simulink model "ddc_bpm_476_066"  (Simulink 7.8)
settings: Solver=ode45  StartTime=0.0  StopTime=0.012  RelTol=1e-3
undefined symbols (not defined in the file): dt_sim, frev_476, Fs_adc, xlipgetpartsetting
libraries: xbsIndex_r4 x601, simulink x5
(part 1 of 6)
settings Model: Creator=lucas.russo  LastModifiedBy=lucas.russo
settings HardwareCC: ProdHWDeviceType=ASIC/FPGA->ASIC/FPGA  TargetIntDivRoundTo=Zero  TargetEndianess=LittleEndian  TargetHWDeviceType=MATLAB Host  ProdEqTarget=off

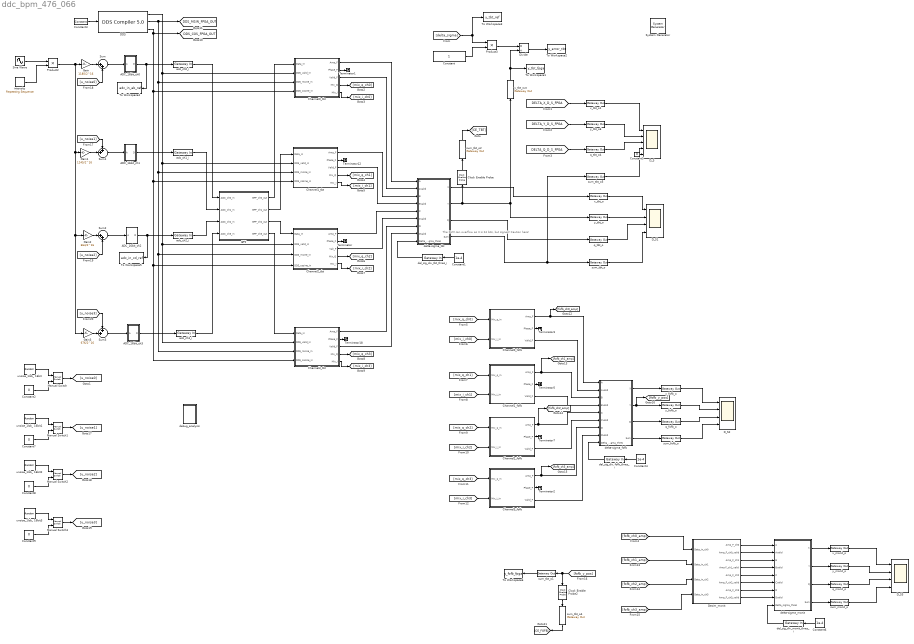
== system ddc_bpm_476_066 ==
  note: The SUM can overflow as it is 24 bits, but signed!
      | Caution here!
  " System Generator" : xbsIndex_r4/ System Generator  Tag=genX  xilinxfamily=virtex6  part=xc6vlx240t  speed=-1  package=ff1156  synthesis_tool=XST  clock_wrapper=Clock Enables  directory=./netlist_ddc_bpm_476_066  proj_type=Project Navigator  Synth_file=XST Defaults  Impl_file=ISE Defaults  testbench=off  simulink_period=dt_sim  sysclk_period=1/Fs_adc*1e9  dcm_input_clock_period=10  incr_netlist=off  trim_vbits=Everywhere in SubSystem  dbl_ovrd=According to Block Masks  core_generation=According to Block Masks  run_coregen=off  deprecated_control=off  eval_field=0  block_type=sysgen
  ADC_16bit_ch0 : Subsystem
  ADC_16bit_ch1 : Subsystem
  ADC_16bit_ch2 : Subsystem
  ADC_16bit_ch3 : Subsystem
  BPF : Subsystem
  Channel0_fofb : Subsystem
  Channel0_tbt : Subsystem
  Channel1_fofb : Subsystem
  Channel1_tbt : Subsystem
  Channel2_fofb : Subsystem
  Channel2_tbt : Subsystem
  Channel3_fofb : Subsystem
  Channel3_tbt : Subsystem
  Clock Enable Probe : xbsIndex_r4/Clock Enable Probe  inherit_constraints=on  block_type=ceprobe
      settings: infoedit="Clock enable extractor.  Produces a Boolean output that mirrors the hardware clock enable associated with the input sample rate.<br><br>Hardware notes: in hardware this block costs nothing."
  Clock Enable Probe2 : xbsIndex_r4/Clock Enable Probe  inherit_constraints=on  block_type=ceprobe
      settings: infoedit="Clock enable extractor.  Produces a Boolean output that mirrors the hardware clock enable associated with the input sample rate.<br><br>Hardware notes: in hardware this block costs nothing."
  Constant : Constant
  Constant1 : Constant  Value=1e-4  OutDataTypeStr=fixdt(1,26,22)
  Constant{2,7..9} (4 alike) : Constant  Value=0  SampleTime=0
  Constant3 : xbsIndex_r4/Constant  const=1  gui_display_data_type=Boolean  arith_type=Boolean  n_bits=24  bin_pt=22  preci_type=Single  exp_width=8  frac_width=24  explicit_period=on  period=dt_sim  equ=P=C  opselect=C  inp2=PCIN>>17  opr=+  inp1=P  carry=CIN  dbl_ovrd=off  block_type=constant
  Constant4 : Constant  Value=1e-4  OutDataTypeStr=fixdt(1,26,22)
  Constant5 : Constant  Value=0
  Constant6 : Constant  Value=1e-4  OutDataTypeStr=fixdt(1,26,22)
  DDS : xbsIndex_r4/DDS Compiler 5.0   partspresent=Phase_Generator_and_SIN_COS_LUT  dds_clock_rate=Fs_adc/1e6  channels=1  parameter_entry=Hardware_Parameters  spurious_free_dynamic_range=36  frequency_resolution=0.4  noise_shaping=Taylor_Series_Corrected  phase_width=30  output_width=24  output_selection=Sine_and_Cosine  negative_sine=on  negative_cosine=off  amplitude_mode=Unit_Circle  memory_type=Auto  optimization_goal=Auto  dsp48_use=Minimal  latency_configuration=Auto  latency=10  has_phase_out=off  has_aclken=off  has_aresetn=off  explicit_period=on  period=dt_sim  data_has_tlast=Not_Required  has_tready=on  s_phase_has_tuser=Not_Required  m_data_has_tuser=Not_Required  m_phase_has_tuser=Not_Required  s_phase_tuser_width=1  s_config_sync_mode=On_Vector  phase_increment=Fixed  output_frequency1=0  output_frequency2=0  output_frequency3=0  output_frequency4=0  output_frequency5=0  output_frequency6=0  output_frequency7=0  output_frequency8=0  output_frequency9=0  output_frequency10=0  output_frequency11=0  output_frequency12=0  output_frequency13=0  output_frequency14=0  output_frequency15=0  output_frequency16=0  pinc1=dds_freq_bin  pinc2='0'  pinc3='0'  pinc4='0'  pinc5='0'  pinc6='0'  pinc7='0'  pinc8='0'  pinc9='0'  pinc10='0'  pinc11='0'  pinc12='0'  pinc13='0'  pinc14='0'  pinc15='0'  pinc16='0'  phase_offset=Fixed  phase_offset_angles1=0  phase_offset_angles2=0  phase_offset_angles3=0  phase_offset_angles4=0  phase_offset_angles5=0  phase_offset_angles6=0  phase_offset_angles7=0  phase_offset_angles8=0  phase_offset_angles9=0  phase_offset_angles10=0  phase_offset_angles11=0  phase_offset_angles12=0  phase_offset_angles13=0  phase_offset_angles14=0  phase_offset_angles15=0  phase_offset_angles16=0  poff1='0'  poff2='0'  poff3='0'  poff4='0'  poff5='0'  poff6='0'  poff7='0'  poff8='0'  poff9='0'  poff10='0'  poff11='0'  poff12='0'  poff13='0'  poff14='0'  poff15='0'  poff16='0'  trim_axipin_name=on  por_mode=false  gui_behaviour=Sysgen  ip_name=DDS Compiler  ip_version=5.0  dsptool_ready=true  wrapper_available=true  port_translation_map={ 'aclken' => 'en', 'aresetn' => 'rst' }  ipcore_xco_need_fpga_part=true  ipcore_fpga_part=xlipgetpartsetting(gcb, {'virtex6', 'xc6vlx75t', '-3', 'ff784'})  ipcore_usecache=true  ipcore_useipmodelcache=true  ipcore_verbose=false  block_type=dds_compiler_v5_0
  D_S : Scope  NumInputPorts=5
      settings: TimeRange=0.0004  YMin=-1~0~10~0~0  YMax=1~0.00025~100~2.5~1  SaveName=ScopeData7  MaxDataPoints=1000000  SampleInput=on
  D_S1 : Scope  NumInputPorts=4
      settings: TimeRange=0.0003  YMin=-1~-1~-1~0.0190031  YMax=1~1~1~0.0210035  SaveName=ScopeData6  MaxDataPoints=1000000  SampleInput=on
  D_S2 : Scope  NumInputPorts=4
      settings: TimeRange=0.002999999999999999  YMin=-1~-1~-1~0.0190031  YMax=1~1~1~0.0210035  SaveName=ScopeData11  MaxDataPoints=1000000  SampleInput=on
  D_S3 : Scope  NumInputPorts=4
      settings: TimeRange=0.0003  YMin=-1~-1~-1~0.0190031  YMax=1~1~1~0.0210035  SaveName=ScopeData12  MaxDataPoints=1000000  SampleInput=on
  Decim_monit : Subsystem
  Divide : Product  Inputs=*/
  Gain : Gain  Gain=1185/2^16
  Gain1 : Gain  Gain=1245/2^16
  Gain2 : Gain  Gain=664/2^16
  Gain3 : Gain  Gain=676/2^16
  Manual Switch{,1..3} (4 alike) : simulink/Signal Routing/Manual Switch  sw=1  action=0  varsize=off
  Product2 : Product  RndMeth=Zero
  Product3 : Product  RndMeth=Zero
  Sine Wave : Sin  Frequency=2*pi*frev_476  SampleTime=0
  Sum : Sum  Inputs=|++
  Sum1 : Sum  Inputs=++|
  Sum2 : Sum  Inputs=|++
  Sum3 : Sum  Inputs=++|
  Terminator{,1..3,5,7,12,18} (8 alike) : Terminator
  To Workspace1 : ToWorkspace  VariableName=y_tbt_fpga  SampleTime=-1  SaveFormat=Structure With Time
      settings: Decimation=35
  To Workspace2 : ToWorkspace  VariableName=y_error_tbt  SampleTime=-1  SaveFormat=Structure With Time
  To Workspace3 : ToWorkspace  VariableName=y_tbt_ref  SampleTime=-1  SaveFormat=Structure With Time
  To Workspace4 : ToWorkspace  VariableName=adc_in_ab_ref  SampleTime=-1  SaveFormat=Structure With Time
  To Workspace5 : ToWorkspace  VariableName=adc_in_cd_ref  SampleTime=-1  SaveFormat=Structure With Time
  To Workspace6 : ToWorkspace  VariableName=y_fofb_fpga  SampleTime=-1  SaveFormat=Structure With Time
      settings: Decimation=R_fofb
  adc_ch0_i : xbsIndex_r4/Gateway In  gui_display_data_type=Fixed-point  arith_type="Signed  (2's comp)"  n_bits=16  bin_pt=15  preci_type=Single  exp_width=8  frac_width=24  quantization=Truncate  overflow=Flag as error  period=dt_sim  dbl_ovrd=off  timing_constraint=None  locs_specified=off  LOCs={}  inherit_from_input=off  UseAsADC=off  ADCChannel='1'  hdl_port=on  block_type=gatewayin
      settings: infoedit="Gateway in block.  Converts inputs of type Simulink integer, single, double and fixed point to  Xilinx fixed-point or floating-point data type.<br><br>Hardware notes:  In hardware these blocks become top level input ports."
  adc_ch1_i : xbsIndex_r4/Gateway In  gui_display_data_type=Fixed-point  arith_type="Signed  (2's comp)"  n_bits=16  bin_pt=15  preci_type=Single  exp_width=8  frac_width=24  quantization=Truncate  overflow=Flag as error  period=dt_sim  dbl_ovrd=off  timing_constraint=None  locs_specified=off  LOCs={}  inherit_from_input=off  UseAsADC=off  ADCChannel='1'  hdl_port=on  block_type=gatewayin
      settings: infoedit="Gateway in block.  Converts inputs of type Simulink integer, single, double and fixed point to  Xilinx fixed-point or floating-point data type.<br><br>Hardware notes:  In hardware these blocks become top level input ports."
  adc_ch2_i : xbsIndex_r4/Gateway In  gui_display_data_type=Fixed-point  arith_type="Signed  (2's comp)"  n_bits=16  bin_pt=15  preci_type=Single  exp_width=8  frac_width=24  quantization=Truncate  overflow=Flag as error  period=dt_sim  dbl_ovrd=off  timing_constraint=None  locs_specified=off  LOCs={}  inherit_from_input=off  UseAsADC=off  ADCChannel='1'  hdl_port=on  block_type=gatewayin
      settings: infoedit="Gateway in block.  Converts inputs of type Simulink integer, single, double and fixed point to  Xilinx fixed-point or floating-point data type.<br><br>Hardware notes:  In hardware these blocks become top level input ports."
  adc_ch3_i : xbsIndex_r4/Gateway In  gui_display_data_type=Fixed-point  arith_type="Signed  (2's comp)"  n_bits=16  bin_pt=15  preci_type=Single  exp_width=8  frac_width=24  quantization=Truncate  overflow=Flag as error  period=dt_sim  dbl_ovrd=off  timing_constraint=None  locs_specified=off  LOCs={}  inherit_from_input=off  UseAsADC=off  ADCChannel='1'  hdl_port=on  block_type=gatewayin
      settings: infoedit="Gateway in block.  Converts inputs of type Simulink integer, single, double and fixed point to  Xilinx fixed-point or floating-point data type.<br><br>Hardware notes:  In hardware these blocks become top level input ports."
  debug_analysis : Subsystem
  del_sig_div_fofb_thres_i : xbsIndex_r4/Gateway In  gui_display_data_type=Fixed-point  arith_type="Signed  (2's comp)"  n_bits=26  bin_pt=22  preci_type=Single  exp_width=8  frac_width=24  quantization=Truncate  overflow=Flag as error  period=dt_sim  dbl_ovrd=off  timing_constraint=Data Rate  locs_specified=off  LOCs={}  inherit_from_input=off  UseAsADC=off  ADCChannel='1'  hdl_port=on  block_type=gatewayin
      settings: infoedit="Gateway in block.  Converts inputs of type Simulink integer, single, double and fixed point to  Xilinx fixed-point or floating-point data type.<br><br>Hardware notes:  In hardware these blocks become top level input ports."
  del_sig_div_monit_thres_i : xbsIndex_r4/Gateway In  gui_display_data_type=Fixed-point  arith_type="Signed  (2's comp)"  n_bits=26  bin_pt=22  preci_type=Single  exp_width=8  frac_width=24  quantization=Truncate  overflow=Flag as error  period=dt_sim  dbl_ovrd=off  timing_constraint=Data Rate  locs_specified=off  LOCs={}  inherit_from_input=off  UseAsADC=off  ADCChannel='1'  hdl_port=on  block_type=gatewayin
      settings: infoedit="Gateway in block.  Converts inputs of type Simulink integer, single, double and fixed point to  Xilinx fixed-point or floating-point data type.<br><br>Hardware notes:  In hardware these blocks become top level input ports."
  del_sig_div_tbt_thres_i : xbsIndex_r4/Gateway In  gui_display_data_type=Fixed-point  arith_type="Signed  (2's comp)"  n_bits=26  bin_pt=22  preci_type=Single  exp_width=8  frac_width=24  quantization=Truncate  overflow=Flag as error  period=dt_sim  dbl_ovrd=off  timing_constraint=Data Rate  locs_specified=off  LOCs={}  inherit_from_input=off  UseAsADC=off  ADCChannel='1'  hdl_port=on  block_type=gatewayin
      settings: infoedit="Gateway in block.  Converts inputs of type Simulink integer, single, double and fixed point to  Xilinx fixed-point or floating-point data type.<br><br>Hardware notes:  In hardware these blocks become top level input ports."
  delta-sigma_fofb : Subsystem
  delta-sigma_monit : Subsystem
  delta-sigma_tbt : Subsystem
  intensity : simulink/Sources/Repeating Sequence  rep_seq_t=[0 1e-4 1e-4 2e-4 2e-4 3e-4 3e-4 4e-4]  rep_seq_y=[1 1 1 1 1 1 1 1]
  q_fofb_o : xbsIndex_r4/Gateway Out  inherit_from_input=on  hdl_port=on  timing_constraint=None  locs_specified=off  LOCs={}  UseAsDAC=off  DACChannel='1'  block_type=gatewayout
      settings: infoedit="Gateway out block.  Converts Xilinx fixed-point or floating-point type inputs into ouputs of type Simulink integer, single, double, or fixed point.<br><br>Hardware notes:  In hardware these blocks become top level output ports or are discarded, depending on how they are configured."
  q_monit_o : xbsIndex_r4/Gateway Out  inherit_from_input=on  hdl_port=on  timing_constraint=None  locs_specified=off  LOCs={}  UseAsDAC=off  DACChannel='1'  block_type=gatewayout
      settings: infoedit="Gateway out block.  Converts Xilinx fixed-point or floating-point type inputs into ouputs of type Simulink integer, single, double, or fixed point.<br><br>Hardware notes:  In hardware these blocks become top level output ports or are discarded, depending on how they are configured."
  q_tbt_o : xbsIndex_r4/Gateway Out  inherit_from_input=on  hdl_port=on  timing_constraint=None  locs_specified=off  LOCs={}  UseAsDAC=off  DACChannel='1'  block_type=gatewayout
      settings: infoedit="Gateway out block.  Converts Xilinx fixed-point or floating-point type inputs into ouputs of type Simulink integer, single, double, or fixed point.<br><br>Hardware notes:  In hardware these blocks become top level output ports or are discarded, depending on how they are configured."
  q_tbt_o4 : xbsIndex_r4/Gateway Out  inherit_from_input=on  hdl_port=off  timing_constraint=None  locs_specified=off  LOCs={}  UseAsDAC=off  DACChannel='1'  block_type=gatewayout
      settings: infoedit="Gateway out block.  Converts Xilinx fixed-point or floating-point type inputs into ouputs of type Simulink integer, single, double, or fixed point.<br><br>Hardware notes:  In hardware these blocks become top level output ports or are discarded, depending on how they are configured."
  sum_fofb_o : xbsIndex_r4/Gateway Out  inherit_from_input=on  hdl_port=on  timing_constraint=None  locs_specified=off  LOCs={}  UseAsDAC=off  DACChannel='1'  block_type=gatewayout
      settings: infoedit="Gateway out block.  Converts Xilinx fixed-point or floating-point type inputs into ouputs of type Simulink integer, single, double, or fixed point.<br><br>Hardware notes:  In hardware these blocks become top level output ports or are discarded, depending on how they are configured."
  sum_monit_o : xbsIndex_r4/Gateway Out  inherit_from_input=on  hdl_port=on  timing_constraint=None  locs_specified=off  LOCs={}  UseAsDAC=off  DACChannel='1'  block_type=gatewayout
      settings: infoedit="Gateway out block.  Converts Xilinx fixed-point or floating-point type inputs into ouputs of type Simulink integer, single, double, or fixed point.<br><br>Hardware notes:  In hardware these blocks become top level output ports or are discarded, depending on how they are configured."
  sum_tbt_o : xbsIndex_r4/Gateway Out  inherit_from_input=on  hdl_port=on  timing_constraint=None  locs_specified=off  LOCs={}  UseAsDAC=off  DACChannel='1'  block_type=gatewayout
      settings: infoedit="Gateway out block.  Converts Xilinx fixed-point or floating-point type inputs into ouputs of type Simulink integer, single, double, or fixed point.<br><br>Hardware notes:  In hardware these blocks become top level output ports or are discarded, depending on how they are configured."
  sum_tbt_o{1..2,4..5} (4 alike) : xbsIndex_r4/Gateway Out  inherit_from_input=on  hdl_port=off  timing_constraint=None  locs_specified=off  LOCs={}  UseAsDAC=off  DACChannel='1'  block_type=gatewayout
      settings: infoedit="Gateway out block.  Converts Xilinx fixed-point or floating-point type inputs into ouputs of type Simulink integer, single, double, or fixed point.<br><br>Hardware notes:  In hardware these blocks become top level output ports or are discarded, depending on how they are configured."
  unoise_1lsb_ 16bit : UniformRandomNumber  Minimum=-0.5*(2/2^16)  Maximum=0.5*(2/2^16)  Seed=49728613  SampleTime=0
  unoise_1lsb_ 16bit1 : UniformRandomNumber  Minimum=-0.5*(2/2^16)  Maximum=0.5*(2/2^16)  Seed=13765948  SampleTime=0
  unoise_1lsb_ 16bit2 : UniformRandomNumber  Minimum=-0.5*(2/2^16)  Maximum=0.5*(2/2^16)  Seed=19875998  SampleTime=0
  unoise_1lsb_ 16bit3 : UniformRandomNumber  Minimum=-0.5*(2/2^16)  Maximum=0.5*(2/2^16)  Seed=367516464  SampleTime=0
  x_fofb_o : xbsIndex_r4/Gateway Out  inherit_from_input=on  hdl_port=on  timing_constraint=None  locs_specified=off  LOCs={}  UseAsDAC=off  DACChannel='1'  block_type=gatewayout
      settings: infoedit="Gateway out block.  Converts Xilinx fixed-point or floating-point type inputs into ouputs of type Simulink integer, single, double, or fixed point.<br><br>Hardware notes:  In hardware these blocks become top level output ports or are discarded, depending on how they are configured."
  x_monit_o : xbsIndex_r4/Gateway Out  inherit_from_input=on  hdl_port=on  timing_constraint=None  locs_specified=off  LOCs={}  UseAsDAC=off  DACChannel='1'  block_type=gatewayout
      settings: infoedit="Gateway out block.  Converts Xilinx fixed-point or floating-point type inputs into ouputs of type Simulink integer, single, double, or fixed point.<br><br>Hardware notes:  In hardware these blocks become top level output ports or are discarded, depending on how they are configured."
  x_tbt_o : xbsIndex_r4/Gateway Out  inherit_from_input=on  hdl_port=on  timing_constraint=None  locs_specified=off  LOCs={}  UseAsDAC=off  DACChannel='1'  block_type=gatewayout
      settings: infoedit="Gateway out block.  Converts Xilinx fixed-point or floating-point type inputs into ouputs of type Simulink integer, single, double, or fixed point.<br><br>Hardware notes:  In hardware these blocks become top level output ports or are discarded, depending on how they are configured."
  x_tbt_o1 : xbsIndex_r4/Gateway Out  inherit_from_input=on  hdl_port=off  timing_constraint=None  locs_specified=off  LOCs={}  UseAsDAC=off  DACChannel='1'  block_type=gatewayout
      settings: infoedit="Gateway out block.  Converts Xilinx fixed-point or floating-point type inputs into ouputs of type Simulink integer, single, double, or fixed point.<br><br>Hardware notes:  In hardware these blocks become top level output ports or are discarded, depending on how they are configured."
  y_fofb_o : xbsIndex_r4/Gateway Out  inherit_from_input=on  hdl_port=on  timing_constraint=None  locs_specified=off  LOCs={}  UseAsDAC=off  DACChannel='1'  block_type=gatewayout
      settings: infoedit="Gateway out block.  Converts Xilinx fixed-point or floating-point type inputs into ouputs of type Simulink integer, single, double, or fixed point.<br><br>Hardware notes:  In hardware these blocks become top level output ports or are discarded, depending on how they are configured."
  y_monit_o : xbsIndex_r4/Gateway Out  inherit_from_input=on  hdl_port=on  timing_constraint=None  locs_specified=off  LOCs={}  UseAsDAC=off  DACChannel='1'  block_type=gatewayout
      settings: infoedit="Gateway out block.  Converts Xilinx fixed-point or floating-point type inputs into ouputs of type Simulink integer, single, double, or fixed point.<br><br>Hardware notes:  In hardware these blocks become top level output ports or are discarded, depending on how they are configured."
  y_tbt_o : xbsIndex_r4/Gateway Out  inherit_from_input=on  hdl_port=on  timing_constraint=None  locs_specified=off  LOCs={}  UseAsDAC=off  DACChannel='1'  block_type=gatewayout
      settings: infoedit="Gateway out block.  Converts Xilinx fixed-point or floating-point type inputs into ouputs of type Simulink integer, single, double, or fixed point.<br><br>Hardware notes:  In hardware these blocks become top level output ports or are discarded, depending on how they are configured."
  y_tbt_o6 : xbsIndex_r4/Gateway Out  inherit_from_input=on  hdl_port=off  timing_constraint=None  locs_specified=off  LOCs={}  UseAsDAC=off  DACChannel='1'  block_type=gatewayout
      settings: infoedit="Gateway out block.  Converts Xilinx fixed-point or floating-point type inputs into ouputs of type Simulink integer, single, double, or fixed point.<br><br>Hardware notes:  In hardware these blocks become top level output ports or are discarded, depending on how they are configured."
  y_tbt_out : xbsIndex_r4/Gateway Out  inherit_from_input=on  hdl_port=off  timing_constraint=None  locs_specified=off  LOCs={}  UseAsDAC=off  DACChannel='1'  block_type=gatewayout
      settings: infoedit="Gateway out block.  Converts Xilinx fixed-point or floating-point type inputs into ouputs of type Simulink integer, single, double, or fixed point.<br><br>Hardware notes:  In hardware these blocks become top level output ports or are discarded, depending on how they are configured."
  tag scope: DDS_COS_FPGA_OUT=global, DDS_MSIN_FPGA_OUT=global
  wires:
  ADC_16bit_ch0/1(D) -> To Workspace4/1, adc_ch0_i/1
  Constant3/1 -> DDS/1
  DDS/1 -> Channel0_tbt/2(DDS_valid_in), Channel2_tbt/2(DDS_valid_in), Channel3_tbt/2(DDS_valid_in), Channel1_tbt/2(DDS_valid_in)
  DDS/2 -> [DDS_MSIN_FPGA_OUT], Channel0_tbt/3(DDS_msine_in), Channel2_tbt/3(DDS_msine_in), Channel3_tbt/3(DDS_msine_in), Channel1_tbt/3(DDS_msine_in)
  DDS/3 -> [DDS_COS_FPGA_OUT], Channel0_tbt/4(DDS_cosine_in), Channel3_tbt/4(DDS_cosine_in), Channel2_tbt/4(DDS_cosine_in), Channel1_tbt/4(DDS_cosine_in)
  ADC_16bit_ch1/1(D) -> adc_ch1_i/1
  ADC_16bit_ch2/1(D) -> To Workspace5/1, adc_ch2_i/1
  ADC_16bit_ch3/1(D) -> adc_ch3_i/1
  Constant/1 -> Product3/2
  Product3/1 -> Divide/1
  Divide/1 -> To Workspace2/1
  [delta_sigma] -> Product3/1, To Workspace3/1
  Channel0_tbt/1(Amp_F) -> delta-sigma_tbt/1(A)
  Channel0_tbt/3(Valid_F) -> delta-sigma_tbt/2(Avalid)
  Channel1_tbt/1(Amp_F) -> delta-sigma_tbt/3(B)
  Channel0_tbt/2(Phase_F) -> Terminator1/1
  Channel2_tbt/3(Vali_F) -> delta-sigma_tbt/6(Cvalid)
  [DELTA_X_D_S_FPGA] -> x_tbt_o1/1
  [DELTA_Y_D_S_FPGA] -> y_tbt_o6/1
  [DELTA_Q_D_S_FPGA] -> q_tbt_o4/1
  x_tbt_o1/1 -> D_S/1
  y_tbt_o6/1 -> D_S/2
  q_tbt_o4/1 -> D_S/3
  sum_tbt_o5/1 -> D_S/4
  x_tbt_o/1 -> D_S1/1
  y_tbt_o/1 -> D_S1/2
  q_tbt_o/1 -> D_S1/3
  sum_tbt_o/1 -> D_S1/4
  delta-sigma_tbt/1(X) -> x_tbt_o/1
  delta-sigma_tbt/2(Y) -> y_tbt_o/1, y_tbt_out/1, Clock Enable Probe/1
  delta-sigma_tbt/3(Q) -> q_tbt_o/1
  delta-sigma_tbt/4(Sum) -> sum_tbt_o/1, sum_tbt_o5/1
  y_tbt_out/1 -> Divide/2, To Workspace1/1
  del_sig_div_tbt_thres_i/1 -> delta-sigma_tbt/9(Delta_sigma_thres)
  Constant1/1 -> del_sig_div_tbt_thres_i/1
  intensity/1 -> Product2/2
  Sine Wave/1 -> Product2/1
  Product2/1 -> Gain2/1, Gain3/1, Gain1/1, Gain/1
  Sum/1 -> ADC_16bit_ch0/1(A)
  Sum1/1 -> ADC_16bit_ch1/1(A)
  Sum2/1 -> ADC_16bit_ch2/1(A)
  Sum3/1 -> ADC_16bit_ch3/1(A)
  unoise_1lsb_ 16bit/1 -> Manual Switch/1
  Constant2/1 -> Manual Switch/2
  Manual Switch/1 -> [u_noise0]
  [u_noise0] -> Sum/2
  [u_noise3] -> Sum3/1
  Channel1_tbt/3(Valid_F) -> delta-sigma_tbt/4(Bvalid)
  Channel3_tbt/1(Amp_F) -> delta-sigma_tbt/7(D)
  Channel3_tbt/3(Valid_F) -> delta-sigma_tbt/8(Dvalid)
  Channel1_tbt/2(Phase_F) -> Terminator12/1
  Channel3_tbt/2(Phase_F) -> Terminator18/1
  Channel0_tbt/4(Mix_Q) -> [mix_q_ch0]
  Channel0_tbt/5(Mix_I) -> [mix_i_ch0]
  Channel1_tbt/4(Mix_Q) -> [mix_q_ch1]
  Channel1_tbt/5(Mix_I) -> [mix_i_ch1]
  Channel2_tbt/4(Mix_Q) -> [mix_q_ch2]
  Channel2_tbt/5(Mix_I) -> [mix_i_ch2]
  Channel3_tbt/4(Mix_Q) -> [mix_q_ch3]
  Channel3_tbt/5(Mix_I) -> [mix_i_ch3]
  [mix_q_ch0] -> Channel0_fofb/1(Mix_q_in)
  [mix_i_ch0] -> Channel0_fofb/2(Mix_i_in)
  [mix_q_ch1] -> Channel1_fofb/1(Mix_q_in)
  [mix_i_ch1] -> Channel1_fofb/2(Mix_i_in)
  [mix_q_ch2] -> Channel2_fofb/1(Mix_q_in)
  [mix_i_ch2] -> Channel2_fofb/2(Mix_i_in)
  [mix_q_ch3] -> Channel3_fofb/1(Mix_q_in)
  [mix_i_ch3] -> Channel3_fofb/2(Mix_i_in)
  del_sig_div_fofb_thres_i/1 -> delta-sigma_fofb/9(Delta_sigma_thres)
  Channel0_fofb/1(Amp_F) -> delta-sigma_fofb/1(A), [fofb_ch0_amp]
  Channel0_fofb/3(Valid_F) -> delta-sigma_fofb/2(Avalid)
  Constant4/1 -> del_sig_div_fofb_thres_i/1
  Channel1_fofb/1(Amp_F) -> delta-sigma_fofb/3(B), [fofb_ch1_amp]
  Channel1_fofb/3(Valid_F) -> delta-sigma_fofb/4(Bvalid)
  Channel2_fofb/1(Amp_F) -> delta-sigma_fofb/5(C), [fofb_ch2_amp]
  Channel2_fofb/3(Valid_F) -> delta-sigma_fofb/6(Cvalid)
  Channel3_fofb/1(Amp_F) -> delta-sigma_fofb/7(D), [fofb_ch3_amp]
  Channel3_fofb/3(Valid_F) -> delta-sigma_fofb/8(Dvalid)
  Channel0_fofb/2(Phase_F) -> Terminator3/1
  Channel1_fofb/2(Phase_F) -> Terminator5/1
  Channel2_fofb/2(Phase_F) -> Terminator7/1
  delta-sigma_fofb/1(X) -> x_fofb_o/1
  delta-sigma_fofb/2(Y) -> y_fofb_o/1, [fofb_y_pos]
  delta-sigma_fofb/3(Q) -> q_fofb_o/1
  delta-sigma_fofb/4(Sum) -> sum_fofb_o/1
  x_fofb_o/1 -> D_S2/1
  y_fofb_o/1 -> D_S2/2
  q_fofb_o/1 -> D_S2/3
  sum_fofb_o/1 -> D_S2/4
  [fofb_ch3_amp] -> Decim_monit/4(Data_in_ch3)
  Constant5/1 -> D_S/5
  [fofb_ch0_amp] -> Decim_monit/1(Data_in_ch0)
  sum_tbt_o1/1 -> To Workspace6/1
  [fofb_y_pos] -> sum_tbt_o1/1, Clock Enable Probe2/1
  [fofb_ch1_amp] -> Decim_monit/2(Data_in_ch1)
  [fofb_ch2_amp] -> Decim_monit/3(Data_in_ch2)
  Channel2_tbt/1(Amp_F) -> delta-sigma_tbt/5(C)
  BPF/1(BPF_ch0_out) -> Channel0_tbt/1(Data_in)
  BPF/2(BPF_ch1_out) -> Channel1_tbt/1(Data_in)
  BPF/3(BPF_ch2_out) -> Channel2_tbt/1(Data_in)
  BPF/4(BPF_ch3_out) -> Channel3_tbt/1(Data_in)
  Channel2_tbt/2(Phase_F) -> Terminator/1
  Channel3_fofb/2(Phase_F) -> Terminator2/1
  adc_ch0_i/1 -> BPF/1(ADC_ch0_in)
  adc_ch1_i/1 -> BPF/2(ADC_ch1_in)
  adc_ch2_i/1 -> BPF/3(ADC_ch2_in)
  adc_ch3_i/1 -> BPF/4(ADC_ch3_in)
  x_monit_o/1 -> D_S3/1
  sum_monit_o/1 -> D_S3/4
  Decim_monit/1(Amp_F_ch0) -> delta-sigma_monit/1(A)
  y_monit_o/1 -> D_S3/2
  q_monit_o/1 -> D_S3/3
  Decim_monit/2(Amp_F_ch0_valid) -> delta-sigma_monit/2(Avalid)
  Decim_monit/3(Amp_F_ch1) -> delta-sigma_monit/3(B)
  Decim_monit/4(Amp F_ch1_valid) -> delta-sigma_monit/4(Bvalid)
  Decim_monit/5(Amp_F_ch2) -> delta-sigma_monit/5(C)
  Decim_monit/6(Amp_F_ch2_valid) -> delta-sigma_monit/6(Cvalid)
  Decim_monit/7(Amp_F_ch3) -> delta-sigma_monit/7(D)
  Decim_monit/8(Amp_F_ch3_valid) -> delta-sigma_monit/8(Dvalid)
  Constant6/1 -> del_sig_div_monit_thres_i/1
  del_sig_div_monit_thres_i/1 -> delta-sigma_monit/9(Delta_sigma_thres)
  delta-sigma_monit/1(X) -> x_monit_o/1
  delta-sigma_monit/2(Y) -> y_monit_o/1
  delta-sigma_monit/3(Q) -> q_monit_o/1
  delta-sigma_monit/4(Sum) -> sum_monit_o/1
  Gain/1 -> Sum/1
  Gain1/1 -> Sum1/2
  Gain2/1 -> Sum2/1
  Gain3/1 -> Sum3/2
  unoise_1lsb_ 16bit1/1 -> Manual Switch1/1
  Constant7/1 -> Manual Switch1/2
  Manual Switch1/1 -> [u_noise1]
  unoise_1lsb_ 16bit2/1 -> Manual Switch2/1
  Constant8/1 -> Manual Switch2/2
  Manual Switch2/1 -> [u_noise2]
  unoise_1lsb_ 16bit3/1 -> Manual Switch3/1
  Constant9/1 -> Manual Switch3/2
  Manual Switch3/1 -> [u_noise3]
  [u_noise1] -> Sum1/1
  [u_noise2] -> Sum2/2
  Clock Enable Probe/1 -> sum_tbt_o2/1
  sum_tbt_o2/1 -> [CE_TBT]
  Clock Enable Probe2/1 -> sum_tbt_o4/1
  sum_tbt_o4/1 -> [CE_FOFB]

== system ddc_bpm_476_066/ADC_16bit_ch0 ==
  A : Inport  OutDataTypeStr=double
  Conversion3 : DataTypeConversion  OutDataTypeStr=fixdt(1,16,2/2^16/1,0/1)  ConvertRealWorld=Stored Integer (SI)  LockScale=on
  Quantizer : Quantizer  QuantizationInterval=1  SampleTime=dt_sim
  Sampler : ZeroOrderHold  SampleTime=1/Fs_adc
  Saturation : Saturate  UpperLimit=65536/2-1  LowerLimit=-65536/2  OutDataTypeStr=Inherit: Inherit via back propagation
  scale : Gain  Gain=2^16/2  SaturateOnIntegerOverflow=on  OutDataTypeStr=Inherit: Same as input  ParamDataTypeStr=Inherit: Same as input
  D : Outport
  wires:
  A/1 -> scale/1
  Conversion3/1 -> D/1
  Quantizer/1 -> Saturation/1
  Sampler/1 -> Quantizer/1
  Saturation/1 -> Conversion3/1
  scale/1 -> Sampler/1

== system ddc_bpm_476_066/ADC_16bit_ch1 ==
  A : Inport  OutDataTypeStr=double
  Conversion3 : DataTypeConversion  OutDataTypeStr=fixdt(1,16,2/2^16/1,0/1)  ConvertRealWorld=Stored Integer (SI)  LockScale=on
  Quantizer : Quantizer  QuantizationInterval=1  SampleTime=dt_sim
  Sampler : ZeroOrderHold  SampleTime=1/Fs_adc
  Saturation : Saturate  UpperLimit=65536/2-1  LowerLimit=-65536/2  OutDataTypeStr=Inherit: Inherit via back propagation
  scale : Gain  Gain=2^16/2  SaturateOnIntegerOverflow=on  OutDataTypeStr=Inherit: Same as input  ParamDataTypeStr=Inherit: Same as input
  D : Outport
  wires:
  A/1 -> scale/1
  Conversion3/1 -> D/1
  Quantizer/1 -> Saturation/1
  Sampler/1 -> Quantizer/1
  Saturation/1 -> Conversion3/1
  scale/1 -> Sampler/1

== system ddc_bpm_476_066/ADC_16bit_ch2 ==
  A : Inport  OutDataTypeStr=double
  Conversion3 : DataTypeConversion  OutDataTypeStr=fixdt(1,16,2/2^16/1,0/1)  ConvertRealWorld=Stored Integer (SI)  LockScale=on
  Quantizer : Quantizer  QuantizationInterval=1  SampleTime=dt_sim
  Sampler : ZeroOrderHold  SampleTime=1/Fs_adc
  Saturation : Saturate  UpperLimit=65536/2-1  LowerLimit=-65536/2  OutDataTypeStr=Inherit: Inherit via back propagation
  scale : Gain  Gain=2^16/2  SaturateOnIntegerOverflow=on  OutDataTypeStr=Inherit: Same as input  ParamDataTypeStr=Inherit: Same as input
  D : Outport
  wires:
  A/1 -> scale/1
  Conversion3/1 -> D/1
  Quantizer/1 -> Saturation/1
  Sampler/1 -> Quantizer/1
  Saturation/1 -> Conversion3/1
  scale/1 -> Sampler/1

== system ddc_bpm_476_066/ADC_16bit_ch3 ==
  A : Inport  OutDataTypeStr=double
  Conversion3 : DataTypeConversion  OutDataTypeStr=fixdt(1,16,2/2^16/1,0/1)  ConvertRealWorld=Stored Integer (SI)  LockScale=on
  Quantizer : Quantizer  QuantizationInterval=1  SampleTime=dt_sim
  Sampler : ZeroOrderHold  SampleTime=1/Fs_adc
  Saturation : Saturate  UpperLimit=65536/2-1  LowerLimit=-65536/2  OutDataTypeStr=Inherit: Inherit via back propagation
  scale : Gain  Gain=2^16/2  SaturateOnIntegerOverflow=on  OutDataTypeStr=Inherit: Same as input  ParamDataTypeStr=Inherit: Same as input
  D : Outport
  wires:
  A/1 -> scale/1
  Conversion3/1 -> D/1
  Quantizer/1 -> Saturation/1
  Sampler/1 -> Quantizer/1
  Saturation/1 -> Conversion3/1
  scale/1 -> Sampler/1

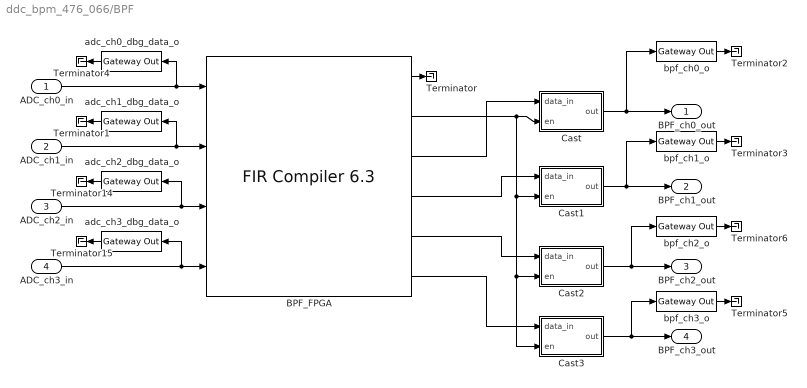
== system ddc_bpm_476_066/BPF ==
  ADC_ch0_in : Inport
  ADC_ch1_in : Inport  Port=2
  ADC_ch2_in : Inport  Port=3
  ADC_ch3_in : Inport  Port=4
  BPF_FPGA : xbsIndex_r4/FIR Compiler 6.3   coefficientvector=Hbpf_adc.Numerator  coefficient_sets=1  coefficient_reload=off  filter_type=Single_Rate  rate_change_type=Integer  interpolation_rate=1  decimation_rate=1  zero_pack_factor=1  channel_sequence=Basic  number_channels=1  pattern_list='P4-0,P4-1,P4-2,P4-3,P4-4'  number_paths=4  ratespecification=Maximum_Possible  sampleperiod=1  hardwareoversamplingrate=1  coefficient_sign=Signed  quantization=Quantize_Only  coefficient_width=16  bestprecision=on  coefficient_fractional_bits=17  coefficient_structure=Inferred  output_rounding_mode=Full_Precision  output_width=34  filter_architecture=Systolic_Multiply_Accumulate  optimization_goal=Area  data_buffer_type=Automatic  coefficient_buffer_type=Automatic  input_buffer_type=Automatic  output_buffer_type=Automatic  preference_for_other_storage=Automatic  multi_column_support=Automatic  columnconfig='29'  inter_column_pipe_length=4  data_has_tlast=Not_Required  m_data_has_tready=off  s_data_has_fifo=off  s_data_has_tuser=Not_Required  m_data_has_tuser=Not_Required  s_config_sync_mode=On_Vector  s_config_method=Single  num_reload_slots=1  has_aclken=off  has_aresetn=off  infoeditControl=ARESETn must be asserted for a minmum of 2 cycles  trim_axipin_name=on  passband_min=0.0  passband_max=0.5  stopband_min=0.5  stopband_max=1.0  filter_selection=1  gui_behaviour=Sysgen_GUI  data_sign=Signed  data_width=16  data_fractional_bits=0  data_tuser_width=1  wrapper_available=true  ip_wrap_arbitrary_binary_point=true  simulation_type=external_xfix  simulation_model=firv6_3_CModel:firv6_3_cmodel  ip_name=FIR Compiler  ip_version=6.3  dsptool_ready=true  ipcore_usecache=true  ipcore_useipmodelcache=true  ipcore_xco_need_fpga_part=true  port_translation_map={ 'aclken' => 'en', 'aresetn' => 'rst' }  run_core_at_system_period=true  ipcore_fpga_part=xlipgetpartsetting(gcb, {'virtex6', 'xc6vlx75t', '-3', 'ff784'})  block_type=fir_compiler_v6_3
      settings: infoedit=Maximum Possible : Maximizes oversampling rate. Abstracted input handshake (no s_data_tvalid) and automatic rate propagation.<br>Hardware Oversampling Rate : Specifies oversampling rate relative to the input sample period. Abstracted input handshake (no s_data_tvalid) and automatic rate propagation.<br>Sample Period : Specifies absolute oversampling rate. No input handshake abstraction (exposes s_data_tvalid) and no rate propagation.
  Cast : Subsystem
  Cast1 : Subsystem
  Cast2 : Subsystem
  Cast3 : Subsystem
  Terminator{,1..6,14..15} (9 alike) : Terminator
  adc_ch0_dbg_data_o : xbsIndex_r4/Gateway Out  inherit_from_input=on  hdl_port=on  timing_constraint=None  locs_specified=off  LOCs={}  UseAsDAC=off  DACChannel='1'  block_type=gatewayout
      settings: infoedit="Gateway out block.  Converts Xilinx fixed-point or floating-point type inputs into ouputs of type Simulink integer, single, double, or fixed point.<br><br>Hardware notes:  In hardware these blocks become top level output ports or are discarded, depending on how they are configured."
  adc_ch1_dbg_data_o : xbsIndex_r4/Gateway Out  inherit_from_input=on  hdl_port=on  timing_constraint=None  locs_specified=off  LOCs={}  UseAsDAC=off  DACChannel='1'  block_type=gatewayout
      settings: infoedit="Gateway out block.  Converts Xilinx fixed-point or floating-point type inputs into ouputs of type Simulink integer, single, double, or fixed point.<br><br>Hardware notes:  In hardware these blocks become top level output ports or are discarded, depending on how they are configured."
  adc_ch2_dbg_data_o : xbsIndex_r4/Gateway Out  inherit_from_input=on  hdl_port=on  timing_constraint=None  locs_specified=off  LOCs={}  UseAsDAC=off  DACChannel='1'  block_type=gatewayout
      settings: infoedit="Gateway out block.  Converts Xilinx fixed-point or floating-point type inputs into ouputs of type Simulink integer, single, double, or fixed point.<br><br>Hardware notes:  In hardware these blocks become top level output ports or are discarded, depending on how they are configured."
  adc_ch3_dbg_data_o : xbsIndex_r4/Gateway Out  inherit_from_input=on  hdl_port=on  timing_constraint=None  locs_specified=off  LOCs={}  UseAsDAC=off  DACChannel='1'  block_type=gatewayout
      settings: infoedit="Gateway out block.  Converts Xilinx fixed-point or floating-point type inputs into ouputs of type Simulink integer, single, double, or fixed point.<br><br>Hardware notes:  In hardware these blocks become top level output ports or are discarded, depending on how they are configured."
  bpf_ch0_o : xbsIndex_r4/Gateway Out  inherit_from_input=on  hdl_port=on  timing_constraint=Data Rate  locs_specified=off  LOCs={}  UseAsDAC=off  DACChannel='1'  block_type=gatewayout
      settings: infoedit="Gateway out block.  Converts Xilinx fixed-point or floating-point type inputs into ouputs of type Simulink integer, single, double, or fixed point.<br><br>Hardware notes:  In hardware these blocks become top level output ports or are discarded, depending on how they are configured."
  bpf_ch1_o : xbsIndex_r4/Gateway Out  inherit_from_input=on  hdl_port=on  timing_constraint=Data Rate  locs_specified=off  LOCs={}  UseAsDAC=off  DACChannel='1'  block_type=gatewayout
      settings: infoedit="Gateway out block.  Converts Xilinx fixed-point or floating-point type inputs into ouputs of type Simulink integer, single, double, or fixed point.<br><br>Hardware notes:  In hardware these blocks become top level output ports or are discarded, depending on how they are configured."
  bpf_ch2_o : xbsIndex_r4/Gateway Out  inherit_from_input=on  hdl_port=on  timing_constraint=Data Rate  locs_specified=off  LOCs={}  UseAsDAC=off  DACChannel='1'  block_type=gatewayout
      settings: infoedit="Gateway out block.  Converts Xilinx fixed-point or floating-point type inputs into ouputs of type Simulink integer, single, double, or fixed point.<br><br>Hardware notes:  In hardware these blocks become top level output ports or are discarded, depending on how they are configured."
  bpf_ch3_o : xbsIndex_r4/Gateway Out  inherit_from_input=on  hdl_port=on  timing_constraint=Data Rate  locs_specified=off  LOCs={}  UseAsDAC=off  DACChannel='1'  block_type=gatewayout
      settings: infoedit="Gateway out block.  Converts Xilinx fixed-point or floating-point type inputs into ouputs of type Simulink integer, single, double, or fixed point.<br><br>Hardware notes:  In hardware these blocks become top level output ports or are discarded, depending on how they are configured."
  BPF_ch0_out : Outport
  BPF_ch1_out : Outport  Port=2
  BPF_ch2_out : Outport  Port=3
  BPF_ch3_out : Outport  Port=4
  wires:
  ADC_ch0_in/1 -> BPF_FPGA/1, adc_ch0_dbg_data_o/1
  ADC_ch1_in/1 -> BPF_FPGA/2, adc_ch1_dbg_data_o/1
  ADC_ch2_in/1 -> BPF_FPGA/3, adc_ch2_dbg_data_o/1
  ADC_ch3_in/1 -> BPF_FPGA/4, adc_ch3_dbg_data_o/1
  BPF_FPGA/3 -> Cast/1(data_in)
  BPF_FPGA/4 -> Cast1/1(data_in)
  BPF_FPGA/5 -> Cast2/1(data_in)
  BPF_FPGA/6 -> Cast3/1(data_in)
  BPF_FPGA/1 -> Terminator/1
  BPF_FPGA/2 -> Cast/2(en), Cast1/2(en), Cast2/2(en), Cast3/2(en)
  Cast/1(out) -> BPF_ch0_out/1, bpf_ch0_o/1
  Cast1/1(out) -> BPF_ch1_out/1, bpf_ch1_o/1
  Cast2/1(out) -> BPF_ch2_out/1, bpf_ch2_o/1
  Cast3/1(out) -> BPF_ch3_out/1, bpf_ch3_o/1
  adc_ch3_dbg_data_o/1 -> Terminator15/1
  adc_ch0_dbg_data_o/1 -> Terminator4/1
  adc_ch1_dbg_data_o/1 -> Terminator1/1
  adc_ch2_dbg_data_o/1 -> Terminator14/1
  bpf_ch0_o/1 -> Terminator2/1
  bpf_ch1_o/1 -> Terminator3/1
  bpf_ch3_o/1 -> Terminator5/1
  bpf_ch2_o/1 -> Terminator6/1

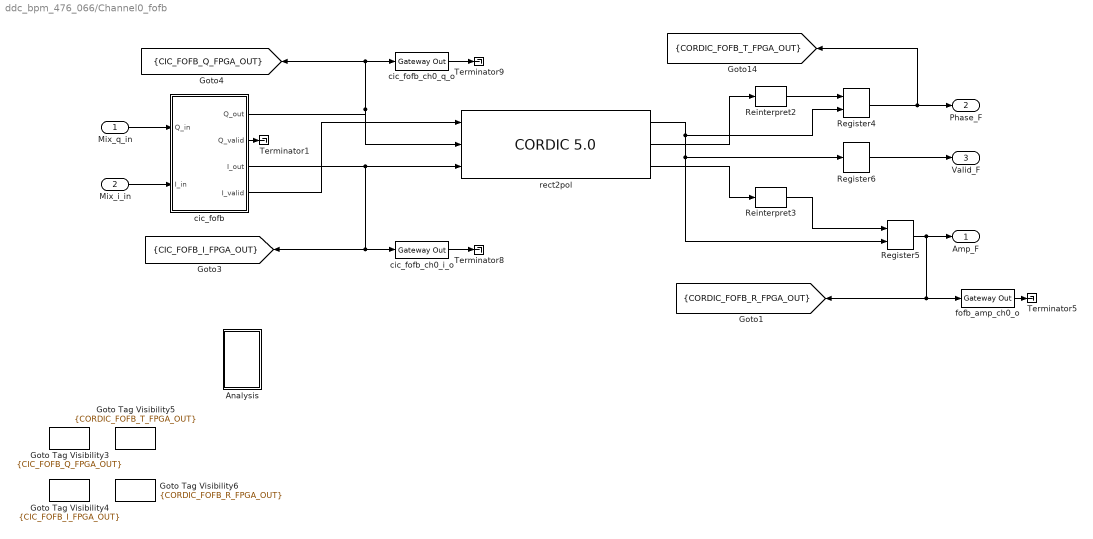
== system ddc_bpm_476_066/Channel0_fofb ==
  Mix_q_in : Inport
  Mix_i_in : Inport  Port=2
  Analysis : Subsystem
  Goto Tag Visibility3 : GotoTagVisibility  GotoTag=CIC_FOFB_Q_FPGA_OUT
  Goto Tag Visibility4 : GotoTagVisibility  GotoTag=CIC_FOFB_I_FPGA_OUT
  Goto Tag Visibility5 : GotoTagVisibility  GotoTag=CORDIC_FOFB_T_FPGA_OUT
  Goto Tag Visibility6 : GotoTagVisibility  GotoTag=CORDIC_FOFB_R_FPGA_OUT
  Register4 : xbsIndex_r4/Register  init=0  rst=off  en=on  dbl_ovrd=off  block_type=register
  Register5 : xbsIndex_r4/Register  init=0  rst=off  en=on  dbl_ovrd=off  block_type=register
  Register6 : xbsIndex_r4/Register  init=0  rst=off  en=off  dbl_ovrd=off  block_type=register
  Reinterpret2 : xbsIndex_r4/Reinterpret  force_arith_type=off  arith_type=Unsigned  force_bin_pt=off  bin_pt=18  block_type=reinterpret
  Reinterpret3 : xbsIndex_r4/Reinterpret  force_arith_type=off  arith_type=Unsigned  force_bin_pt=off  bin_pt=19  block_type=reinterpret
  Terminator{1,5,8..9} (4 alike) : Terminator
  cic_fofb : Subsystem
  cic_fofb_ch0_i_o : xbsIndex_r4/Gateway Out  inherit_from_input=on  hdl_port=on  timing_constraint=Data Rate  locs_specified=off  LOCs={}  UseAsDAC=off  DACChannel='1'  block_type=gatewayout
      settings: infoedit="Gateway out block.  Converts Xilinx fixed-point or floating-point type inputs into ouputs of type Simulink integer, single, double, or fixed point.<br><br>Hardware notes:  In hardware these blocks become top level output ports or are discarded, depending on how they are configured."
  cic_fofb_ch0_q_o : xbsIndex_r4/Gateway Out  inherit_from_input=on  hdl_port=on  timing_constraint=Data Rate  locs_specified=off  LOCs={}  UseAsDAC=off  DACChannel='1'  block_type=gatewayout
      settings: infoedit="Gateway out block.  Converts Xilinx fixed-point or floating-point type inputs into ouputs of type Simulink integer, single, double, or fixed point.<br><br>Hardware notes:  In hardware these blocks become top level output ports or are discarded, depending on how they are configured."
  fofb_amp_ch0_o : xbsIndex_r4/Gateway Out  inherit_from_input=on  hdl_port=on  timing_constraint=Data Rate  locs_specified=off  LOCs={}  UseAsDAC=off  DACChannel='1'  block_type=gatewayout
      settings: infoedit="Gateway out block.  Converts Xilinx fixed-point or floating-point type inputs into ouputs of type Simulink integer, single, double, or fixed point.<br><br>Hardware notes:  In hardware these blocks become top level output ports or are discarded, depending on how they are configured."
  rect2pol : xbsIndex_r4/CORDIC 5.0   functional_selection=Translate  architectural_configuration=Parallel  pipelining_mode=Maximum  data_format=SignedFraction  phase_format=Radians  input_width=24  output_width=24  round_mode=Nearest_Even  iterations=0  precision=36  compensation_scaling=BRAM  coarse_rotation=on  aclken=off  aresetn=off  out_tready=off  cartesian_has_tuser=off  cartesian_has_tlast=off  cartesian_tuser_width=1  phase_has_tuser=off  phase_has_tlast=off  phase_tuser_width=1  out_tlast_behv=Null  flow_control=NonBlocking  optimize_goal=Resources  trim_axipin_name=on  ip_name=CORDIC  ip_version=5.0  dsptool_ready=true  ipcore_usecache=true  ipcore_useipmodelcache=true  wrapper_available=true  port_translation_map={ 'aclken' => 'en', 'aresetn' => 'rst' }  block_type=cordic_v5_0
      settings: infoedit=CORDIC 5.0
  Amp_F : Outport
  Phase_F : Outport  Port=2
  Valid_F : Outport  Port=3
  tag scope: CIC_FOFB_I_FPGA_OUT=scoped, CIC_FOFB_Q_FPGA_OUT=scoped, CORDIC_FOFB_R_FPGA_OUT=scoped, CORDIC_FOFB_T_FPGA_OUT=scoped
  wires:
  cic_fofb/3(I_out) -> rect2pol/3, cic_fofb_ch0_i_o/1, [CIC_FOFB_I_FPGA_OUT]
  cic_fofb/1(Q_out) -> [CIC_FOFB_Q_FPGA_OUT], cic_fofb_ch0_q_o/1, rect2pol/2
  cic_fofb/2(Q_valid) -> Terminator1/1
  rect2pol/1 -> Register4/2, Register5/2, Register6/1
  rect2pol/2 -> Reinterpret2/1
  rect2pol/3 -> Reinterpret3/1
  Register4/1 -> Phase_F/1, [CORDIC_FOFB_T_FPGA_OUT]
  Register5/1 -> Amp_F/1, [CORDIC_FOFB_R_FPGA_OUT], fofb_amp_ch0_o/1
  Register6/1 -> Valid_F/1
  Reinterpret2/1 -> Register4/1
  Reinterpret3/1 -> Register5/1
  fofb_amp_ch0_o/1 -> Terminator5/1
  cic_fofb_ch0_q_o/1 -> Terminator9/1
  cic_fofb_ch0_i_o/1 -> Terminator8/1
  Mix_q_in/1 -> cic_fofb/1(Q_in)
  Mix_i_in/1 -> cic_fofb/2(I_in)
  cic_fofb/4(I_valid) -> rect2pol/1

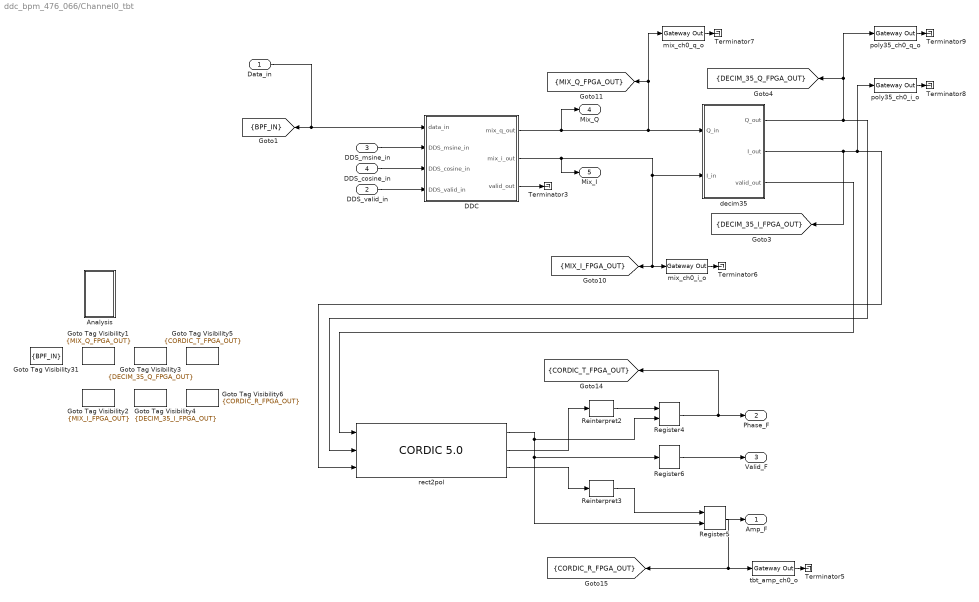
== system ddc_bpm_476_066/Channel0_tbt ==
  Data_in : Inport
  DDS_valid_in : Inport  Port=2
  DDS_msine_in : Inport  Port=3
  DDS_cosine_in : Inport  Port=4
  Analysis : Subsystem
  DDC : Subsystem
  Goto Tag Visibility1 : GotoTagVisibility  GotoTag=MIX_Q_FPGA_OUT
  Goto Tag Visibility2 : GotoTagVisibility  GotoTag=MIX_I_FPGA_OUT
  Goto Tag Visibility3 : GotoTagVisibility  GotoTag=DECIM_35_Q_FPGA_OUT
  Goto Tag Visibility31 : GotoTagVisibility  GotoTag=BPF_IN
  Goto Tag Visibility4 : GotoTagVisibility  GotoTag=DECIM_35_I_FPGA_OUT
  Goto Tag Visibility5 : GotoTagVisibility  GotoTag=CORDIC_T_FPGA_OUT
  Goto Tag Visibility6 : GotoTagVisibility  GotoTag=CORDIC_R_FPGA_OUT
  Register4 : xbsIndex_r4/Register  init=0  rst=off  en=on  dbl_ovrd=off  block_type=register
  Register5 : xbsIndex_r4/Register  init=0  rst=off  en=on  dbl_ovrd=off  block_type=register
  Register6 : xbsIndex_r4/Register  init=0  rst=off  en=off  dbl_ovrd=off  block_type=register
  Reinterpret2 : xbsIndex_r4/Reinterpret  force_arith_type=off  arith_type=Unsigned  force_bin_pt=off  bin_pt=18  block_type=reinterpret
  Reinterpret3 : xbsIndex_r4/Reinterpret  force_arith_type=off  arith_type=Unsigned  force_bin_pt=off  bin_pt=19  block_type=reinterpret
  Terminator{3,5..9} (6 alike) : Terminator
  decim35 : Subsystem
  mix_ch0_i_o : xbsIndex_r4/Gateway Out  inherit_from_input=on  hdl_port=on  timing_constraint=Data Rate  locs_specified=off  LOCs={}  UseAsDAC=off  DACChannel='1'  block_type=gatewayout
      settings: infoedit="Gateway out block.  Converts Xilinx fixed-point or floating-point type inputs into ouputs of type Simulink integer, single, double, or fixed point.<br><br>Hardware notes:  In hardware these blocks become top level output ports or are discarded, depending on how they are configured."
  mix_ch0_q_o : xbsIndex_r4/Gateway Out  inherit_from_input=on  hdl_port=on  timing_constraint=Data Rate  locs_specified=off  LOCs={}  UseAsDAC=off  DACChannel='1'  block_type=gatewayout
      settings: infoedit="Gateway out block.  Converts Xilinx fixed-point or floating-point type inputs into ouputs of type Simulink integer, single, double, or fixed point.<br><br>Hardware notes:  In hardware these blocks become top level output ports or are discarded, depending on how they are configured."
  poly35_ch0_i_o : xbsIndex_r4/Gateway Out  inherit_from_input=on  hdl_port=on  timing_constraint=Data Rate  locs_specified=off  LOCs={}  UseAsDAC=off  DACChannel='1'  block_type=gatewayout
      settings: infoedit="Gateway out block.  Converts Xilinx fixed-point or floating-point type inputs into ouputs of type Simulink integer, single, double, or fixed point.<br><br>Hardware notes:  In hardware these blocks become top level output ports or are discarded, depending on how they are configured."
  poly35_ch0_q_o : xbsIndex_r4/Gateway Out  inherit_from_input=on  hdl_port=on  timing_constraint=Data Rate  locs_specified=off  LOCs={}  UseAsDAC=off  DACChannel='1'  block_type=gatewayout
      settings: infoedit="Gateway out block.  Converts Xilinx fixed-point or floating-point type inputs into ouputs of type Simulink integer, single, double, or fixed point.<br><br>Hardware notes:  In hardware these blocks become top level output ports or are discarded, depending on how they are configured."
  rect2pol : xbsIndex_r4/CORDIC 5.0   functional_selection=Translate  architectural_configuration=Parallel  pipelining_mode=Maximum  data_format=SignedFraction  phase_format=Radians  input_width=24  output_width=24  round_mode=Nearest_Even  iterations=0  precision=36  compensation_scaling=BRAM  coarse_rotation=on  aclken=off  aresetn=off  out_tready=off  cartesian_has_tuser=off  cartesian_has_tlast=off  cartesian_tuser_width=1  phase_has_tuser=off  phase_has_tlast=off  phase_tuser_width=1  out_tlast_behv=Null  flow_control=NonBlocking  optimize_goal=Resources  trim_axipin_name=on  ip_name=CORDIC  ip_version=5.0  dsptool_ready=true  ipcore_usecache=true  ipcore_useipmodelcache=true  wrapper_available=true  port_translation_map={ 'aclken' => 'en', 'aresetn' => 'rst' }  block_type=cordic_v5_0
      settings: infoedit=CORDIC 5.0
  tbt_amp_ch0_o : xbsIndex_r4/Gateway Out  inherit_from_input=on  hdl_port=on  timing_constraint=Data Rate  locs_specified=off  LOCs={}  UseAsDAC=off  DACChannel='1'  block_type=gatewayout
      settings: infoedit="Gateway out block.  Converts Xilinx fixed-point or floating-point type inputs into ouputs of type Simulink integer, single, double, or fixed point.<br><br>Hardware notes:  In hardware these blocks become top level output ports or are discarded, depending on how they are configured."
  Amp_F : Outport
  Phase_F : Outport  Port=2
  Valid_F : Outport  Port=3
  Mix_Q : Outport  Port=4
  Mix_I : Outport  Port=5
  tag scope: BPF_IN=scoped, CORDIC_R_FPGA_OUT=scoped, CORDIC_T_FPGA_OUT=scoped, DECIM_35_I_FPGA_OUT=scoped, DECIM_35_Q_FPGA_OUT=scoped, MIX_I_FPGA_OUT=scoped, MIX_Q_FPGA_OUT=scoped
  wires:
  Data_in/1 -> [BPF_IN], DDC/1(data_in)
  DDC/2(mix_i_out) -> decim35/2(I_in), [MIX_I_FPGA_OUT], mix_ch0_i_o/1, Mix_I/1
  DDC/3(valid_out) -> Terminator3/1
  DDC/1(mix_q_out) -> decim35/1(Q_in), [MIX_Q_FPGA_OUT], mix_ch0_q_o/1, Mix_Q/1
  decim35/2(I_out) -> [DECIM_35_I_FPGA_OUT], rect2pol/3, poly35_ch0_i_o/1
  decim35/1(Q_out) -> rect2pol/2, [DECIM_35_Q_FPGA_OUT], poly35_ch0_q_o/1
  decim35/3(valid_out) -> rect2pol/1
  rect2pol/1 -> Register4/2, Register5/2, Register6/1
  rect2pol/2 -> Reinterpret2/1
  rect2pol/3 -> Reinterpret3/1
  Register4/1 -> Phase_F/1, [CORDIC_T_FPGA_OUT]
  Register5/1 -> Amp_F/1, [CORDIC_R_FPGA_OUT], tbt_amp_ch0_o/1
  Register6/1 -> Valid_F/1
  Reinterpret2/1 -> Register4/1
  Reinterpret3/1 -> Register5/1
  tbt_amp_ch0_o/1 -> Terminator5/1
  mix_ch0_i_o/1 -> Terminator6/1
  mix_ch0_q_o/1 -> Terminator7/1
  poly35_ch0_q_o/1 -> Terminator9/1
  poly35_ch0_i_o/1 -> Terminator8/1
  DDS_valid_in/1 -> DDC/4(DDS_valid_in)
  DDS_msine_in/1 -> DDC/2(DDS_msine_in)
  DDS_cosine_in/1 -> DDC/3(DDS_cosine_in)
